simulink model "Cartesian_nonlinear_controler"  (R2022a)
settings: Solver=VariableStepAuto  StartTime=0.0  StopTime=50  RelTol=1e-3
settings Model: PauseTimes=2  Creator=18222  LastModifiedBy=18222
settings DebuggingCC: UnderSpecifiedDimensionMsg=warning

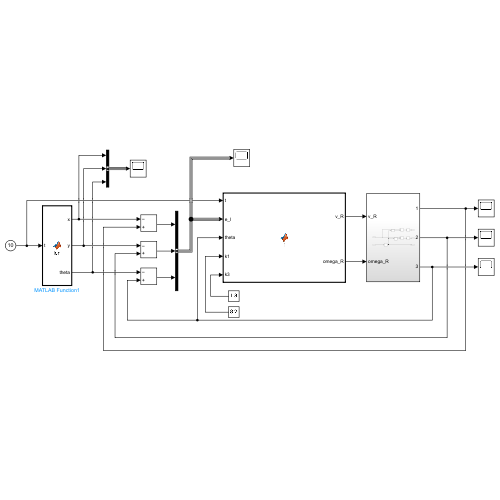
[thumbnail: Simulink's stored preview of the top-level diagram]
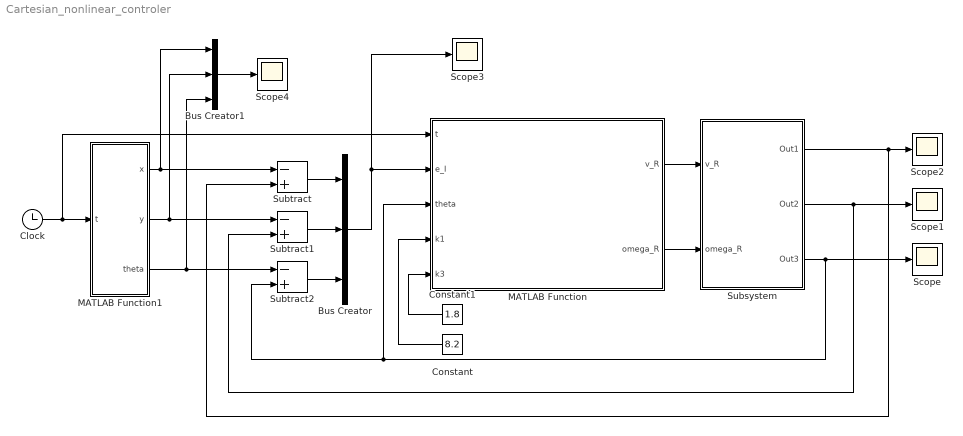
== system Cartesian_nonlinear_controler ==
  Bus Creator : BusCreator  Inputs=3
  Bus Creator1 : BusCreator  Inputs=3
  Clock : Clock
  Constant : Constant  Value=8.2
  Constant1 : Constant  Value=1.8
  MATLAB Function : MATLAB Function  TreatAsAtomicUnit=on
  MATLAB Function1 : MATLAB Function  TreatAsAtomicUnit=on
  Scope{,1..4} (5 alike) : Scope
  Subsystem : Subsystem
  Subtract : Sum  Inputs=-+
  Subtract1 : Sum  Inputs=-+
  Subtract2 : Sum  Inputs=-+
  wires:
  MATLAB Function1/1(x) -> Bus Creator1/1, Subtract/1
  MATLAB Function1/2(y) -> Bus Creator1/2, Subtract1/1
  MATLAB Function1/3(theta) -> Bus Creator1/3, Subtract2/1
  Subtract/1 -> Bus Creator/1
  Subtract1/1 -> Bus Creator/2
  Subtract2/1 -> Bus Creator/3
  Clock/1 -> MATLAB Function1/1(t), MATLAB Function/1(t)
  Subsystem/3(Out3) -> Scope/1, MATLAB Function/3(theta), Subtract2/2
  Subsystem/1(Out1) -> Scope2/1, Subtract/2
  Subsystem/2(Out2) -> Scope1/1, Subtract1/2
  MATLAB Function/1(v_R) -> Subsystem/1(v_R)
  MATLAB Function/2(omega_R) -> Subsystem/2(omega_R)
  Constant/1 -> MATLAB Function/4(k1)
  Constant1/1 -> MATLAB Function/5(k3)
  Bus Creator/1 -> Scope3/1, MATLAB Function/2(e_I)
  Bus Creator1/1 -> Scope4/1

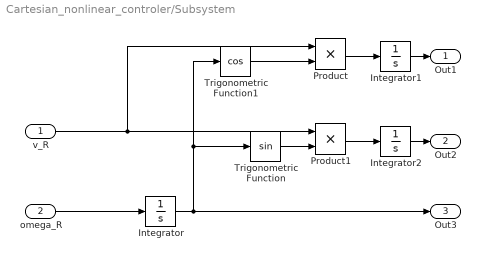
== system Cartesian_nonlinear_controler/Subsystem ==
  v_R : Inport
  omega_R : Inport  Port=2
  Integrator : Integrator
  Integrator1 : Integrator
  Integrator2 : Integrator
  Product : Product
  Product1 : Product
  Trigonometric Function : Trigonometry
  Trigonometric Function1 : Trigonometry  Operator=cos
  Out1 : Outport
  Out2 : Outport  Port=2
  Out3 : Outport  Port=3
  wires:
  v_R/1 -> Product/1, Product1/1
  Integrator2/1 -> Out2/1
  Integrator/1 -> Trigonometric Function/1, Trigonometric Function1/1, Out3/1
  Product/1 -> Integrator1/1
  omega_R/1 -> Integrator/1
  Trigonometric Function/1 -> Product1/2
  Product1/1 -> Integrator2/1
  Trigonometric Function1/1 -> Product/2
  Integrator1/1 -> Out1/1

== matlab function Cartesian_nonlinear_controler/MATLAB Function1 ==
  data: x output; t input; y output; theta output
function [x, y, theta] = target(t)

%定点控制
x=15;
y=10;
theta=0.2;

== matlab function Cartesian_nonlinear_controler/MATLAB Function ==
  data: t input; v_R output size=1; e_I input; theta input; omega_R output size=1; k1 input; k3 input
function [v_R,omega_R] = model(t,e_I,theta,k1,k3)

ex_I = e_I(1);
ey_I = e_I(2);
etheta_I = e_I(3);

%坐标系变换
e_R=[cos(theta),sin(theta),0;
    sin(theta),cos(theta),0;
    0, 0, 1]*[ex_I;ey_I;etheta_I];

%控制器
v_R=-k1*e_R(1);
omega_R=e_R(2)^2*sin(t)-k3*e_R(3);
